simulink model "doubletank_linear"  (R2019a)
settings: Solver=VariableStepAuto  StartTime=0.0  StopTime=500  RelTol=1e-3
values from neighbouring files (symbols this model uses):
  K = 5    [doubletank.m]    (also in fcn.m; kalman_dynamic.m; kalman_dynamic_EKF.m; kalman_f_stationary.m)
  T = 35    [doubletank.m]    (also in fcn.m; kalman_dynamic.m; kalman_dynamic_EKF.m; kalman_f_stationary.m)
settings Model: Creator=lukkar-4  LastModifiedBy=lukkar-4

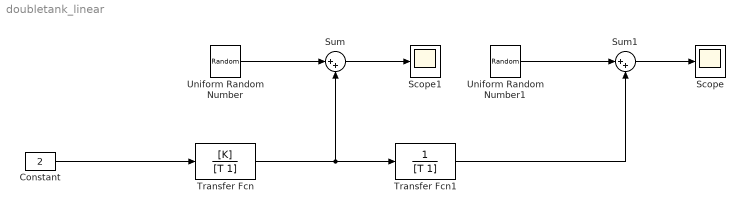
== system doubletank_linear ==
  Constant : Constant  Value=2
  Scope : Scope
  Scope1 : Scope
  Sum : Sum  Inputs=|++
  Sum1 : Sum  Inputs=|++
  Transfer Fcn : TransferFcn  Numerator=[K]  Denominator=[T 1]
  Transfer Fcn1 : TransferFcn  Denominator=[T 1]
  Uniform Random Number : UniformRandomNumber  Minimum=-0.1  Maximum=0.1  SampleTime=0.1
  Uniform Random Number1 : UniformRandomNumber  Minimum=-0.1  Maximum=0.1  SampleTime=0.1
  wires:
  Constant/1 -> Transfer Fcn/1
  Transfer Fcn/1 -> Sum/2, Transfer Fcn1/1
  Sum/1 -> Scope1/1
  Uniform Random Number/1 -> Sum/1
  Transfer Fcn1/1 -> Sum1/2
  Uniform Random Number1/1 -> Sum1/1
  Sum1/1 -> Scope/1
